simulink model "Demo_veDYNA_cs"  (Simulink 7.6)
settings: Solver=ode1  StartTime=0  StopTime=15  FixedStep=1/500  RelTol=1e-3
model workspace (MAT data in the model file):
  mbox_table : struct (value not decoded)
  model_closed = 0
  sim_status = 0
PreLoadFcn:
  | PreScanveDYNAPreLoadFcn(bdroot);
  | check_NUTS_defined;
  | 
  | assignin('base',['model_closed_' bdroot],false);
PostLoadFcn:
  | PreScanveDYNAPostLoadFcn(bdroot);
  | 
InitFcn:
  | vdy_SetExternalInputSource('ManLongCtrl',1,'Brake','other');
  | vdy_SetExternalInputSource('ManLongCtrl',1,'EngineTorque','other');
  | vdy_SetExternalInputSource('ManLatCtrl',1,'Steering','other');
  | 
  | PreScanveDYNAInitFcn(bdroot);
  | PreScanExperimentInitFcn(bdroot)
StopFcn:
  | PreScanExperimentStopFcn(bdroot)
undefined symbols (not defined in the file): at_period, CPT, vm_at_pulsewidth, vm_driver_dflt_gain, x_ini_VRML, y_ini_VRML, z_ini_VRML
libraries: dyna_cpt_lib x93, simulink x16, simulink_extras x14, PreScanSimulinkLibrary x6, anilib x3, dyna_lib x3, dyna_manctrl_lib x2, dyna_road_lib x2, PreScanUsefulBlocks x1, dyna_io_lib x1, dyna_demo_lib x1, dyna_usr_maneuver_states_lib x1
(part 1 of 8)
CloseFcn:
  | evalin('base',['clear model_closed_' bdroot]);
settings Model: TDMajorMDLVersion=3  TDMinorMDLVersion=3  TDMDLPatchlevel=0  Creator=PRESCAN  LastModifiedBy=cappend  BufferReuse=off
settings OptimizationCC: BlockReduction=off  BooleanDataType=off  ConditionallyExecuteInputs=off  OptimizeBlockIOStorage=off  BufferReuse=off  ExpressionFolding=off  LocalBlockOutputs=off  InitFltsAndDblsToZero=on
settings DebuggingCC: SaveWithParameterizedLinksMsg=none  SignalResolutionControl=TryResolveAllWithWarning  MultiTaskDSMMsg=warning  MultiTaskCondExecSysMsg=none  StrictBusMsg=Warning
settings RTWCC: IncludeERTFirstTime=on
settings GRTTargetCC: TargetFcnLib=ansi_tfl_tmw.mat

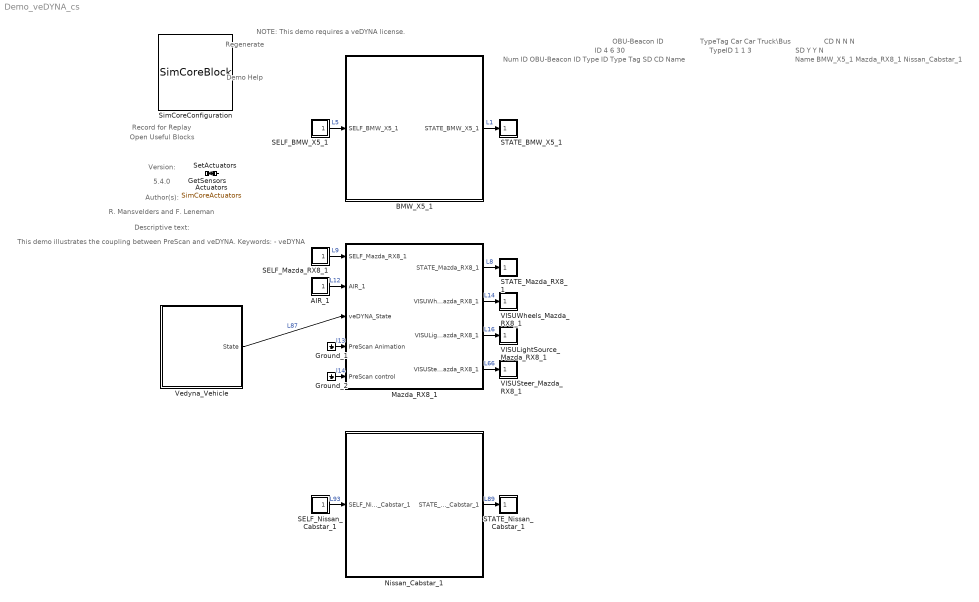
== system Demo_veDYNA_cs ==
  note: Demo Help
  note: NOTE: This demo requires a veDYNA license.
  note: Regenerate
  note: Record for Replay
  note: Open Useful Blocks
  note: Version:
  note: 5.4.0
  note: Author(s):
  note: R. Mansvelders and F. Leneman
  note: Descriptive text:
  note: This demo illustrates the
      | coupling between PreScan and
      | veDYNA.
      |
      | Keywords:
      | - veDYNA
  note: ID
      |
      | 4
      | 6
      | 30
  note: OBU-Beacon ID
  note: TypeID
      |
      | 1
      | 1
      | 3
  note: TypeTag
      |
      | Car
      | Car
      | Truck\Bus
  note: SD
      |
      | Y
      | Y
      | N
  note: CD
      |
      | N
      | N
      | N
  note: Name
      |
      | BMW_X5_1
      | Mazda_RX8_1
      | Nissan_Cabstar_1
  note: Num ID OBU-Beacon ID Type ID Type Tag SD CD Name
  AIR_1 : Subsystem  Tag=AIR  mask(PreScan Source Block: Actor Independent Receiver (AIR)){Angle=60, Range=75, NrEntitiesOut=1, PortName=AIR_1, PortIndex=16, PortWidth=6, TimeStep=1/500}
      mask prompts: Angle "User Specified: Angle [deg]"; Range "User Specified: Range [m]"; NrEntitiesOut "Auto-Assigned: # of Visible Actors in Experiment [-]"; PortName "Auto-Assigned: Port Name [-]"; PortIndex "Auto-Assigned: Port Index [-]"; PortWidth "Auto-Assigned: Port Dimensions [-]"; TimeStep "Auto-Assigned: Upload Period [s]"
      mask help:
      | The Actor Information Receiver sensor provides a fast, simple and generic detection solution which is not tied up to a specific technology. The AIR detects the intersection point of the bounding box with the straight line from the sensor axis system to the middle of the bounding box.
      |
      | For more information, please click Help.
      settings: DeleteFcn=PreScanBlockDeleteFcn;
      mask Help: eval('openHelp(413)')
      mask Display: image(imread('AIR.png'))
  Actuators : DataStoreMemory  Tag=Actuators  DataStoreName=SimCoreActuators  InitialValue=zeros(289,1)
      settings: DeleteFcn=PreScanBlockDeleteFcn;
  BMW_X5_1 : Subsystem  Tag=WorldObjectSubSystem  InitFcn=UniqueId = '15';
      mask Display: image(imread('BMW_X5.jpg'));color('white');text(0,0,' ID=4\n')
  GetSensors : Subsystem  Tag=GetSensors  mask(PreScan Simulation Core Block){NrOfSensors=30, TimeStep=1/500}
      mask prompts: NrOfSensors "Number of sensor values"; TimeStep "Timestep [s]"
      mask help:
      | Please do not remove this block from the PreScan compilation sheet,
      | as it contains essential configuration parameters for a PreScan simulation.
      settings: DeleteFcn=PreScanBlockDeleteFcn;
  Ground_1 : Ground
  Ground_2 : Ground
  Mazda_RX8_1 : Subsystem  Tag=WorldObjectSubSystem  InitFcn=UniqueId = '17';
      mask Display: image(imread('Mazda_RX8.jpg'));color('white');text(0,0,' ID=6\n')
  Nissan_Cabstar_1 : Subsystem  Tag=WorldObjectSubSystem  InitFcn=UniqueId = '45';
      mask Display: image(imread('Nissan_Cabstar.jpg'));color('white');text(0,0,' ID=30\n')
  SELF_BMW_X5_1 : Subsystem  Tag=SELF  mask(PreScan Source Block: SELF){PortName=SELF_BMW_X5_1, PortIndex=0, PortWidth=8, TimeStep=1/500}
      mask prompts: PortName "Auto-Assigned: Port Name [-]"; PortIndex "Auto-Assigned: Port Index [-]"; PortWidth "Auto-Assigned: Port Dimensions"; TimeStep "Auto-Assigned: Upload Period [s]"
      mask help:
      | The SELF port shows (state) information of the actor itself. The outputs are position in the experiment's axis system and the GPS coordinates, and the object's absolute velocity and compass heading.
      |
      | For more information, please click Help.
      settings: DeleteFcn=PreScanBlockDeleteFcn;
      mask Help: eval('openHelp(462)')
      mask Display: image(imread('GPS.png'))
  SELF_Mazda_RX8_1 : Subsystem  Tag=SELF  mask(PreScan Source Block: SELF){PortName=SELF_Mazda_RX8_1, PortIndex=8, PortWidth=8, TimeStep=1/500}
      mask prompts: PortName "Auto-Assigned: Port Name [-]"; PortIndex "Auto-Assigned: Port Index [-]"; PortWidth "Auto-Assigned: Port Dimensions"; TimeStep "Auto-Assigned: Upload Period [s]"
      mask help:
      | The SELF port shows (state) information of the actor itself. The outputs are position in the experiment's axis system and the GPS coordinates, and the object's absolute velocity and compass heading.
      |
      | For more information, please click Help.
      settings: DeleteFcn=PreScanBlockDeleteFcn;
      mask Help: eval('openHelp(462)')
      mask Display: image(imread('GPS.png'))
  SELF_Nissan_Cabstar_1 : Subsystem  Tag=SELF  mask(PreScan Source Block: SELF){PortName=SELF_Nissan_Cabstar_1, PortIndex=22, PortWidth=8, TimeStep=1/500}
      mask prompts: PortName "Auto-Assigned: Port Name [-]"; PortIndex "Auto-Assigned: Port Index [-]"; PortWidth "Auto-Assigned: Port Dimensions"; TimeStep "Auto-Assigned: Upload Period [s]"
      mask help:
      | The SELF port shows (state) information of the actor itself. The outputs are position in the experiment's axis system and the GPS coordinates, and the object's absolute velocity and compass heading.
      |
      | For more information, please click Help.
      settings: DeleteFcn=PreScanBlockDeleteFcn;
      mask Help: eval('openHelp(462)')
      mask Display: image(imread('GPS.png'))
  STATE_BMW_X5_1 : Subsystem  Tag=State  mask(PreScan Sink Block: State){x0=10.1045246, y0=47.3258, z0=0.69, Roll0=0, Pitch0=0, Yaw0=0, override=off, Mode=Positioning}
      mask prompts: x0 "Ini x-position VEHICLE wrt GLOBAL axis system [m]"; y0 "Ini y-position VEHICLE wrt GLOBAL axis system [m]"; z0 "Ini z-position VEHICLE wrt GLOBAL axis system [m]"; Roll0 "Ini roll-angle BODY wrt VEHICLE axis system [rad]"; Pitch0 "Ini pitch-angle BODY wrt VEHICLE axis system [rad]"; Yaw0 "Ini yaw-angle VEHICLE wrt GLOBAL axis system [rad]"; override "Override Mode"
      mask help:
      | The Actor State contains a vector signal of size (9x1), containing the following signals:
      |
      | -  Position                  (x,y,z)                                     [m]
      | -  Velocity                  (vx,vy,vz)                               [m/s]
      | -  Angles                    (Roll, Pitch, Yaw)                   [rad]
      |
      | The Actor state is defined in the global axis system.
      | The state is superponed on the Initial position defined in the GUI.
      |
      | For more information, please click Help.
      settings: DeleteFcn=PreScanBlockDeleteFcn;
      mask Help: eval('openHelp(222)')
      mask StyleString: edit,edit,edit,edit,edit,edit,checkbox,popup(Positioning|Dynamics)
      mask CallbackString: ||||||StateOverrideFcn('General')|
      mask Display: image(imread('State.png'))
  STATE_Mazda_RX8_1 : Subsystem  Tag=State  mask(PreScan Sink Block: State){x0=-9.892563, y0=51.9277153, z0=0.51, Roll0=0, Pitch0=0, Yaw0=0, override=on, Mode=Positioning}
      mask prompts: x0 "Ini x-position VEHICLE wrt GLOBAL axis system [m]"; y0 "Ini y-position VEHICLE wrt GLOBAL axis system [m]"; z0 "Ini z-position VEHICLE wrt GLOBAL axis system [m]"; Roll0 "Ini roll-angle BODY wrt VEHICLE axis system [rad]"; Pitch0 "Ini pitch-angle BODY wrt VEHICLE axis system [rad]"; Yaw0 "Ini yaw-angle VEHICLE wrt GLOBAL axis system [rad]"; override "Override Mode"
      mask help:
      | The Actor State contains a vector signal of size (9x1), containing the following signals:
      |
      | -  Position                  (x,y,z)                                     [m]
      | -  Velocity                  (vx,vy,vz)                               [m/s]
      | -  Angles                    (Roll, Pitch, Yaw)                   [rad]
      |
      | The Actor state is defined in the global axis system.
      | The state is superponed on the Initial position defined in the GUI.
      |
      | For more information, please click Help.
      settings: DeleteFcn=PreScanBlockDeleteFcn;
      mask Help: eval('openHelp(222)')
      mask StyleString: edit,edit,edit,edit,edit,edit,checkbox,popup(Positioning|Dynamics)
      mask CallbackString: ||||||StateOverrideFcn('General')|
      mask Display: image(imread('State.png'))
  STATE_Nissan_Cabstar_1 : Subsystem  Tag=State  mask(PreScan Sink Block: State){x0=-14, y0=47.3258, z0=0.88, Roll0=0, Pitch0=0, Yaw0=0, override=off, Mode=Positioning}
      mask prompts: x0 "Ini x-position VEHICLE wrt GLOBAL axis system [m]"; y0 "Ini y-position VEHICLE wrt GLOBAL axis system [m]"; z0 "Ini z-position VEHICLE wrt GLOBAL axis system [m]"; Roll0 "Ini roll-angle BODY wrt VEHICLE axis system [rad]"; Pitch0 "Ini pitch-angle BODY wrt VEHICLE axis system [rad]"; Yaw0 "Ini yaw-angle VEHICLE wrt GLOBAL axis system [rad]"; override "Override Mode"
      mask help:
      | The Actor State contains a vector signal of size (9x1), containing the following signals:
      |
      | -  Position                  (x,y,z)                                     [m]
      | -  Velocity                  (vx,vy,vz)                               [m/s]
      | -  Angles                    (Roll, Pitch, Yaw)                   [rad]
      |
      | The Actor state is defined in the global axis system.
      | The state is superponed on the Initial position defined in the GUI.
      |
      | For more information, please click Help.
      settings: DeleteFcn=PreScanBlockDeleteFcn;
      mask Help: eval('openHelp(222)')
      mask StyleString: edit,edit,edit,edit,edit,edit,checkbox,popup(Positioning|Dynamics)
      mask CallbackString: ||||||StateOverrideFcn('General')|
      mask Display: image(imread('State.png'))
  SetActuators : Subsystem  Tag=SetActuators  mask(PreScan Simulation Core Block){TimeStep=1/500, NrOfActuators=289}
      mask prompts: TimeStep "Timestep [s]"; NrOfActuators "Number of actuator values"
      mask help:
      | Please do not remove this block from the PreScan compilation sheet,
      | as it contains essential configuration parameters for a PreScan simulation.
      settings: DeleteFcn=PreScanBlockDeleteFcn;
  SimCoreConfiguration : M-S-Function  Tag=SimCoreConfiguration  Description=A17A9ED9750FB4A86C3BBE414AD268275C76F333D22CB9730EAC2D9853BCC9CB  FunctionName=SimCoreBlock  Parameters=ExperimentXML PortsXML SimulationCore HostName CheckStart EnableLog RfR  mask(PreScan Simulation Core Configurator){SimulationCore=NUTS, HostName=0, CheckStart=0, prescanversion='5.4.0', EnableLog=off, RfR=0}
      mask prompts: SimulationCore "Simulation Core"; HostName "Simulation Host"; CheckStart "Show START Dialog"; prescanversion "PreScan Version"; EnableLog "Create TA Log"; RfR "Record for Replay"
      mask help:
      | Please do not remove this block from the PreScan compilation sheet,
      | as it contains essential configuration parameter for a PreScan simulation.
      mask init:
      | model = bdroot;
      | ExperimentXML = [model(1:end-3) '.pex'];
      | PortsXML = [model '_ports.pcd'];
      settings: DeleteFcn=PreScanBlockDeleteFcn;  ModelCloseFcn=assignin('base',['model_closed_' bdroot],true);
      mask Display: image(imread('prescanlogo.ico'))
  VISULightSource_Mazda_RX8_1 : Subsystem  Tag=VisuLightSource
      settings: DeleteFcn=PreScanBlockDeleteFcn;
      mask Type: PreScan Sink Block: VisuLightSource
      mask Description:
      | The VisuLightSource block provides a way to animate Light Sources of the indicator, braking, fog and main lights of a vehicle.
      | 
      | For more information, please click Help.
      mask Help: eval('openHelp(223)')
      mask Display: image(imread('RearLight.png'))
  VISUSteer_Mazda_RX8_1 : Subsystem  Tag=VisuSteer
      settings: DeleteFcn=PreScanBlockDeleteFcn;
      mask Type: PreScan Sink Block: VisuSteer
      mask Description:
      | The VisuSteer block provides a way to adapt the orientation of the steering column and steering wheel of a vehicle.
      | 
      | For more information, please click Help.
      mask Help: eval('openHelp(223)')
      mask Display: image(imread('steeringwheel.png'))
  VISUWheels_Mazda_RX8_1 : Subsystem  Tag=VisuWheels
      settings: DeleteFcn=PreScanBlockDeleteFcn;
      mask Type: PreScan Sink Block: VisuWheels
      mask Description:
      | The VisuWheels block provides a way to animate the wheels of a vehicle, with steering, rotation (because of velocity) and z-displacement.
      | 
      | For more information, please click Help.
      mask Help: eval('openHelp(223)')
      mask Display: image(imread('wheel.png'))
  Vedyna_Vehicle : Subsystem  Tag=UserSpecified_Subsys  Description=C:\Program Files\DYNAwareR3.3\work.current\models\vedyna_vehicle.mdl  mask(User specified subsystem){update=off, sourcefilename=C:\\Program Files\\DYNAwareR3.3\\work.current\\models\\vedyna_vehicle.mdl}
      mask prompts: update "Update (default: not checked)"; sourcefilename "Source file name"
      mask help:
      | A User-specified model may be selected as Controller or Dynamics of the vehicle. PreScan will copy the contents of the User-specified model into the user-specified model block.
      |
      | If update checkbox is checked the current user-specified model block will be deleted and will be REPLACED by (new) user specified model blocks. So, the current user specified model elements will be lost.
      |
      | Warning: If a new user-specified model is selected in the GUI, the user-specified model will be replaced.
      settings: DeleteFcn=PreScanBlockDeleteFcn;
      mask Help: eval('openHelp(227)')
      mask Display:
      | image(imread('UserSpecDyn.png'))
      | port_label('output', 1, 'State'); text(0,0,' veDYNA Vehicle\n')
  wires:
  SetActuators/1(dummy) -> GetSensors/1(dummy)
  BMW_X5_1/1(STATE_BMW_X5_1) -> STATE_BMW_X5_1/1(State)  "L1"
  SELF_BMW_X5_1/1(U) -> BMW_X5_1/1(SELF_BMW_X5_1)  "L5"
  Mazda_RX8_1/1(STATE_Mazda_RX8_1) -> STATE_Mazda_RX8_1/1(State)  "L8"
  SELF_Mazda_RX8_1/1(U) -> Mazda_RX8_1/1(SELF_Mazda_RX8_1)  "L9"
  AIR_1/1(U) -> Mazda_RX8_1/2(AIR_1)  "L12"
  Mazda_RX8_1/2(VISUWheels_Mazda_RX8_1) -> VISUWheels_Mazda_RX8_1/1(Wheels)  "L14"
  Mazda_RX8_1/3(VISULightSource_Mazda_RX8_1) -> VISULightSource_Mazda_RX8_1/1(Lights)  "L16"
  Mazda_RX8_1/4(VISUSteer_Mazda_RX8_1) -> VISUSteer_Mazda_RX8_1/1(Steer)  "L66"
  Vedyna_Vehicle/1(State) -> Mazda_RX8_1/3(veDYNA_State)  "L87"
  Nissan_Cabstar_1/1(STATE_Nissan_Cabstar_1) -> STATE_Nissan_Cabstar_1/1(State)  "L89"
  SELF_Nissan_Cabstar_1/1(U) -> Nissan_Cabstar_1/1(SELF_Nissan_Cabstar_1)  "L93"
  Ground_1/1 -> Mazda_RX8_1/4(PreScan Animation)  "l13"
  Ground_2/1 -> Mazda_RX8_1/5(PreScan control)  "l14"

== system Demo_veDYNA_cs/AIR_1 ==
  Selector : Selector  IndexMode=Zero-based  IndexOptions=Starting index (dialog)  Indices=PortIndex  OutputSizes=PortWidth(1)
  U : Outport
  wires:
  Selector/1 -> U/1
  [SimCoreSensors] -> Selector/1

== system Demo_veDYNA_cs/BMW_X5_1 ==
  SELF_BMW_X5_1 : Inport  Tag=SELFInport
  SELF_Demux : Subsystem  Tag=DemuxSELF
      settings: DeleteFcn=PreScanBlockDeleteFcn;
      mask Type: PreScan Demux Block:
      mask Display:
      | port_label('output',1,'x [m]')
      | port_label('output',2,'y [m]')
      | port_label('output',3,'z [m]','texmode','on')
      | port_label('output',4,'Rotx [deg]','texmode','on')
      | port_label('output',5,'Roty [deg]','texmode','on')
      | port_label('output',6,'Rotz [deg]','texmode','on')
      | port_label('output',7,'GPS lat [deg]','texmode','on')
      | port_label('output',8,'GPS long [deg]','texmode','on')
      | port_label('output',9,'GPS alt [m]','texmode','on')
      | port_label('output',10,'Velocity [m/s]')
      | port_label('output',11,'Heading [deg]')
      | port_label('output',12,'Yaw rate [deg/s]')
  Terminator_{1..12} (12 alike) : Terminator
  Trajectories : Subsystem  Tag=Trajectories
      settings: DeleteFcn=PreScanBlockDeleteFcn;
      mask Display: image(imread('Trajectory.png'));
  STATE_BMW_X5_1 : Outport  Tag=StateOutport
  wires:
  SELF_BMW_X5_1/1 -> SELF_Demux/1(SELF)  "L6"
  Trajectories/1(State) -> STATE_BMW_X5_1/1  "L7"
  SELF_Demux/1(x [m]) -> Terminator_1/1  "l1"
  SELF_Demux/2(y [m]) -> Terminator_2/1  "l2"
  SELF_Demux/3(z [m]) -> Terminator_3/1  "l3"
  SELF_Demux/4(rotx [deg]) -> Terminator_4/1  "l4"
  SELF_Demux/5(roty [deg]) -> Terminator_5/1  "l5"
  SELF_Demux/6(rotz [deg]) -> Terminator_6/1  "l6"
  SELF_Demux/7(GPS lat [deg]) -> Terminator_7/1  "l7"
  SELF_Demux/8(GPS long [deg]) -> Terminator_8/1  "l8"
  SELF_Demux/9(GPS alt [m]) -> Terminator_9/1  "l9"
  SELF_Demux/10(velocity [m/s]) -> Terminator_10/1  "l10"
  SELF_Demux/11(heading [deg]) -> Terminator_11/1  "l11"
  SELF_Demux/12(yaw rate [deg/s]) -> Terminator_12/1  "l12"

== system Demo_veDYNA_cs/GetSensors ==
  dummy : Inport
  GetSensors : M-S-Function  FunctionName=GetSensorsBlock  Parameters=TimeStep, NrOfSensors
      mask Type: PreScan GetSensors block
      mask Description: Reads new sensor values from the simulation core
  tag scope: SimCoreSensors=global
  wires:
  GetSensors/1 -> [SimCoreSensors]
  dummy/1 -> GetSensors/1

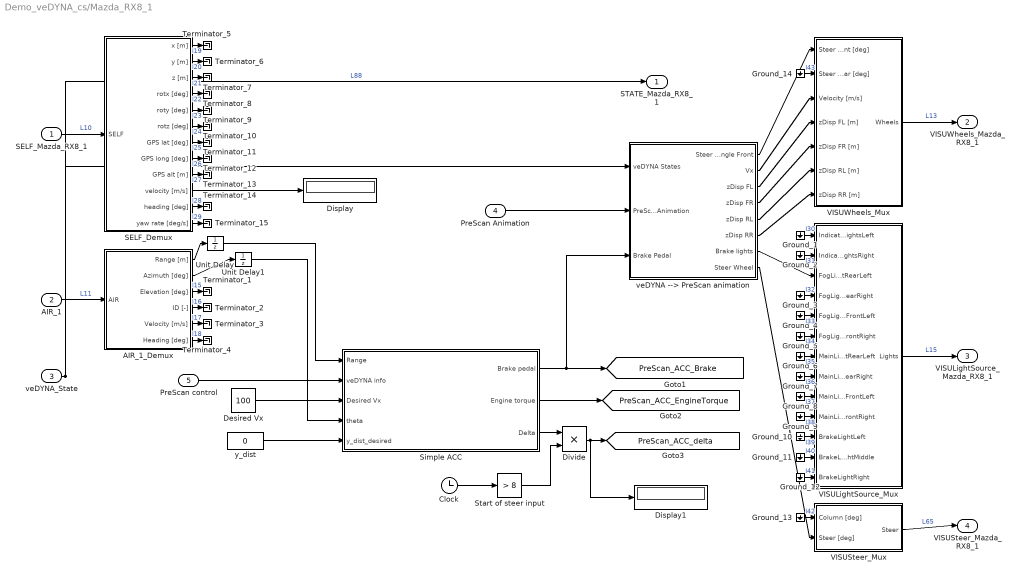
== system Demo_veDYNA_cs/Mazda_RX8_1 ==
  SELF_Mazda_RX8_1 : Inport  Tag=SELFInport
  AIR_1 : Inport  Tag=AIRInport  Port=2
  veDYNA_State : Inport  Tag=veDYNA_StateInport  Port=3
  PreScan Animation : Inport  Tag=AIRInport  Port=4
  PreScan control : Inport  Tag=AIRInport  Port=5
  AIR_1_Demux : Subsystem  Tag=DemuxAIR  mask(PreScan Demux Block:){DetectionType=BBox}
      mask prompts: DetectionType "Detection Type"
      mask init:
      | switch DetectionType
      |     case 1
      |         DetectionTypeStr = 'Shortest';
      |     case 2
      |         DetectionTypeStr = 'BBox';
      |     case 3
      |         DetectionTypeStr = 'CoG';
      |     otherwise
      |         DetectionTypeStr = 'Unknown';
      | end
      settings: DeleteFcn=PreScanBlockDeleteFcn;
      mask StyleString: popup(Shortest|BBox|CoG)
      mask Display:
      | disp(char('Det. type:         ',['{\it',DetectionTypeStr,'}']),'texmode','on')
      | port_label('output',1,'Range [m]')
      | port_label('output',2,'{\theta} [deg]','texmode','on')
      | port_label('output',3,'{\phi} [deg]','texmode','on')
      | port_label('output',4,'ID [-]','texmode','on')
      | port_label('output',5,'Velocity [m/s]','texmode','on')
      | port_label('output',6,'Heading [deg]','texmode','on')
  Clock : Clock
      settings: Decimation=10
  Desired Vx : Constant  Value=100
  Display : Display
  Display1 : Display
  Divide : Product  Inputs=**
  Ground_{1..14} (14 alike) : Ground
  SELF_Demux : Subsystem  Tag=DemuxSELF
      settings: DeleteFcn=PreScanBlockDeleteFcn;
      mask Type: PreScan Demux Block:
      mask Display:
      | port_label('output',1,'x [m]')
      | port_label('output',2,'y [m]')
      | port_label('output',3,'z [m]','texmode','on')
      | port_label('output',4,'Rotx [deg]','texmode','on')
      | port_label('output',5,'Roty [deg]','texmode','on')
      | port_label('output',6,'Rotz [deg]','texmode','on')
      | port_label('output',7,'GPS lat [deg]','texmode','on')
      | port_label('output',8,'GPS long [deg]','texmode','on')
      | port_label('output',9,'GPS alt [m]','texmode','on')
      | port_label('output',10,'Velocity [m/s]')
      | port_label('output',11,'Heading [deg]')
      | port_label('output',12,'Yaw rate [deg/s]')
  Simple ACC : Subsystem
  Start of steer input : simulink/Logic and Bit Operations/Compare To Constant  SystemSampleTime=-1  relop=>  const=8  LogicOutDataTypeMode=uint8  ZeroCross=off
  Terminator_{1..15} (15 alike) : Terminator
  Unit Delay : UnitDelay  SampleTime=-1
  Unit Delay1 : UnitDelay  SampleTime=-1
  VISULightSource_Mux : Subsystem  Tag=MuxLightSource
      settings: DeleteFcn=PreScanBlockDeleteFcn;
      mask Type: PreScan Mux Block:
  VISUSteer_Mux : Subsystem  Tag=MuxSteer
      settings: DeleteFcn=PreScanBlockDeleteFcn;
      mask Type: PreScan Mux Block:
  VISUWheels_Mux : Subsystem  Tag=MuxWheels
      settings: DeleteFcn=PreScanBlockDeleteFcn;
      mask Type: PreScan Mux Block:
  veDYNA --> PreScan animation : Subsystem
  y_dist : Constant  Value=0
  STATE_Mazda_RX8_1 : Outport  Tag=StateOutport
  VISUWheels_Mazda_RX8_1 : Outport  Tag=VisuWheelsOutport  Port=2
  VISULightSource_Mazda_RX8_1 : Outport  Tag=VisuLightsOutport  Port=3
  VISUSteer_Mazda_RX8_1 : Outport  Tag=VisuSteerOutport  Port=4
  tag scope: PreScan_ACC_Brake=global, PreScan_ACC_EngineTorque=global, PreScan_ACC_delta=global
  wires:
  Desired Vx/1 -> Simple ACC/3(Desired Vx)
  y_dist/1 -> Simple ACC/5(y_dist_desired)
  Simple ACC/3(Delta) -> Divide/1
  Simple ACC/1(Brake pedal) -> [PreScan_ACC_Brake], veDYNA --> PreScan animation/3(Brake Pedal)
  Simple ACC/2(Engine torque) -> [PreScan_ACC_EngineTorque]
  Unit Delay/1 -> Simple ACC/1(Range)
  Unit Delay1/1 -> Simple ACC/4(theta)
  Divide/1 -> [PreScan_ACC_delta], Display1/1
  Clock/1 -> Start of steer input/1
  Start of steer input/1 -> Divide/2
  veDYNA_State/1 -> veDYNA --> PreScan animation/1(veDYNA States), STATE_Mazda_RX8_1/1  "L88"
  veDYNA --> PreScan animation/8(Steer Wheel) -> VISUSteer_Mux/2(Steer [deg])
  AIR_1_Demux/1(Range [m]) -> Unit Delay/1
  AIR_1_Demux/2(Azimuth [deg]) -> Unit Delay1/1
  PreScan control/1 -> Simple ACC/2(veDYNA info)
  SELF_Demux/10(velocity [m/s]) -> Display/1
  PreScan Animation/1 -> veDYNA --> PreScan animation/2(PreScan Animation)
  veDYNA --> PreScan animation/1(Steer Angle Front) -> VISUWheels_Mux/1(Steer Angle Front [deg])
  veDYNA --> PreScan animation/2(Vx) -> VISUWheels_Mux/3(Velocity [m/s])
  veDYNA --> PreScan animation/3(zDisp FL) -> VISUWheels_Mux/4(zDisp FL [m])
  veDYNA --> PreScan animation/4(zDisp FR) -> VISUWheels_Mux/5(zDisp FR [m])
  veDYNA --> PreScan animation/5(zDisp RL) -> VISUWheels_Mux/6(zDisp RL [m])
  veDYNA --> PreScan animation/6(zDisp RR) -> VISUWheels_Mux/7(zDisp RR [m])
  veDYNA --> PreScan animation/7(Brake lights) -> VISULightSource_Mux/3(FogLightRearLeft)
  SELF_Mazda_RX8_1/1 -> SELF_Demux/1(SELF)  "L10"
  AIR_1/1 -> AIR_1_Demux/1(AIR)  "L11"
  VISUWheels_Mux/1(Wheels) -> VISUWheels_Mazda_RX8_1/1  "L13"
  VISULightSource_Mux/1(Lights) -> VISULightSource_Mazda_RX8_1/1  "L15"
  VISUSteer_Mux/1(Steer) -> VISUSteer_Mazda_RX8_1/1  "L65"
  AIR_1_Demux/3(Elevation [deg]) -> Terminator_1/1  "l15"
  AIR_1_Demux/4(ID [-]) -> Terminator_2/1  "l16"
  AIR_1_Demux/5(Velocity [m/s]) -> Terminator_3/1  "l17"
  AIR_1_Demux/6(Heading [deg]) -> Terminator_4/1  "l18"
  SELF_Demux/1(x [m]) -> Terminator_5/1  "l19"
  SELF_Demux/2(y [m]) -> Terminator_6/1  "l20"
  SELF_Demux/3(z [m]) -> Terminator_7/1  "l21"
  SELF_Demux/4(rotx [deg]) -> Terminator_8/1  "l22"
  SELF_Demux/5(roty [deg]) -> Terminator_9/1  "l23"
  SELF_Demux/6(rotz [deg]) -> Terminator_10/1  "l24"
  SELF_Demux/7(GPS lat [deg]) -> Terminator_11/1  "l25"
  SELF_Demux/8(GPS long [deg]) -> Terminator_12/1  "l26"
  SELF_Demux/9(GPS alt [m]) -> Terminator_13/1  "l27"
  SELF_Demux/11(heading [deg]) -> Terminator_14/1  "l28"
  SELF_Demux/12(yaw rate [deg/s]) -> Terminator_15/1  "l29"
  Ground_1/1 -> VISULightSource_Mux/1(IndicatorLightsLeft)  "l30"
  Ground_2/1 -> VISULightSource_Mux/2(IndicatorLightsRight)  "l31"
  Ground_3/1 -> VISULightSource_Mux/4(FogLightRearRight)  "l32"
  Ground_4/1 -> VISULightSource_Mux/5(FogLightFrontLeft)  "l33"
  Ground_5/1 -> VISULightSource_Mux/6(FogLightFrontRight)  "l34"
  Ground_6/1 -> VISULightSource_Mux/7(MainLightRearLeft)  "l35"
  Ground_7/1 -> VISULightSource_Mux/8(MainLightRearRight)  "l36"
  Ground_8/1 -> VISULightSource_Mux/9(MainLightFrontLeft)  "l37"
  Ground_9/1 -> VISULightSource_Mux/10(MainLightFrontRight)  "l38"
  Ground_10/1 -> VISULightSource_Mux/11(BrakeLightLeft)  "l39"
  Ground_11/1 -> VISULightSource_Mux/12(BrakeLightMiddle)  "l40"
  Ground_12/1 -> VISULightSource_Mux/13(BrakeLightRight)  "l41"
  Ground_13/1 -> VISUSteer_Mux/1(Column [deg])  "l42"
  Ground_14/1 -> VISUWheels_Mux/2(Steer Angle Rear [deg])  "l43"

== system Demo_veDYNA_cs/Nissan_Cabstar_1 ==
  SELF_Nissan_Cabstar_1 : Inport  Tag=SELFInport
  SELF_Demux : Subsystem  Tag=DemuxSELF
      settings: DeleteFcn=PreScanBlockDeleteFcn;
      mask Type: PreScan Demux Block:
      mask Display:
      | port_label('output',1,'x [m]')
      | port_label('output',2,'y [m]')
      | port_label('output',3,'z [m]','texmode','on')
      | port_label('output',4,'Rotx [deg]','texmode','on')
      | port_label('output',5,'Roty [deg]','texmode','on')
      | port_label('output',6,'Rotz [deg]','texmode','on')
      | port_label('output',7,'GPS lat [deg]','texmode','on')
      | port_label('output',8,'GPS long [deg]','texmode','on')
      | port_label('output',9,'GPS alt [m]','texmode','on')
      | port_label('output',10,'Velocity [m/s]')
      | port_label('output',11,'Heading [deg]')
      | port_label('output',12,'Yaw rate [deg/s]')
  Terminator_{1..12} (12 alike) : Terminator
  Trajectories : Subsystem  Tag=Trajectories
      settings: DeleteFcn=PreScanBlockDeleteFcn;
      mask Display: image(imread('Trajectory.png'));
  STATE_Nissan_Cabstar_1 : Outport  Tag=StateOutport
  wires:
  SELF_Nissan_Cabstar_1/1 -> SELF_Demux/1(SELF)  "L94"
  Trajectories/1(State) -> STATE_Nissan_Cabstar_1/1  "L95"
  SELF_Demux/1(x [m]) -> Terminator_1/1  "l44"
  SELF_Demux/2(y [m]) -> Terminator_2/1  "l45"
  SELF_Demux/3(z [m]) -> Terminator_3/1  "l46"
  SELF_Demux/4(rotx [deg]) -> Terminator_4/1  "l47"
  SELF_Demux/5(roty [deg]) -> Terminator_5/1  "l48"
  SELF_Demux/6(rotz [deg]) -> Terminator_6/1  "l49"
  SELF_Demux/7(GPS lat [deg]) -> Terminator_7/1  "l50"
  SELF_Demux/8(GPS long [deg]) -> Terminator_8/1  "l51"
  SELF_Demux/9(GPS alt [m]) -> Terminator_9/1  "l52"
  SELF_Demux/10(velocity [m/s]) -> Terminator_10/1  "l53"
  SELF_Demux/11(heading [deg]) -> Terminator_11/1  "l54"
  SELF_Demux/12(yaw rate [deg/s]) -> Terminator_12/1  "l55"

== system Demo_veDYNA_cs/SELF_BMW_X5_1 ==
  Selector : Selector  IndexMode=Zero-based  IndexOptions=Starting index (dialog)  Indices=PortIndex  OutputSizes=PortWidth(1)
  U : Outport
  wires:
  Selector/1 -> U/1
  [SimCoreSensors] -> Selector/1

== system Demo_veDYNA_cs/SELF_Mazda_RX8_1 ==
  Selector : Selector  IndexMode=Zero-based  IndexOptions=Starting index (dialog)  Indices=PortIndex  OutputSizes=PortWidth(1)
  U : Outport
  wires:
  Selector/1 -> U/1
  [SimCoreSensors] -> Selector/1

== system Demo_veDYNA_cs/SELF_Nissan_Cabstar_1 ==
  Selector : Selector  IndexMode=Zero-based  IndexOptions=Starting index (dialog)  Indices=PortIndex  OutputSizes=PortWidth(1)
  U : Outport
  wires:
  Selector/1 -> U/1
  [SimCoreSensors] -> Selector/1

== system Demo_veDYNA_cs/STATE_BMW_X5_1 ==
  State : Inport
  Acceleration : Subsystem  mask(ToSensorWorld){PortName=Acceleration_BMW_X5_1, PortIndex=6, PortWidth=3, TimeStep=1/500}
      mask prompts: PortName "Port Name [-]"; PortIndex "Index [-]"; PortWidth "Port Dimensions [-]"; TimeStep "Upload Period [s]"
      mask help: Sends signal(s) from Simulink to the Sensor World
      mask Help:
      | Sends signal(s) from Simulink to the Sensor World.
      | 
      | - Port Name [-]: specifies the name of the output terminal of the Simulink block.
      | - Index [-]: specifies the start position in the output vector sent to the Sensor World
      | - Port dimensions [-]: specifies the width (number of scalars) of the output port
      | - Upload period [s]: specifies the upload period (in seconds) of the port.
      mask Display: port_label('input', 1, PortName)
  Demux : Demux  Outputs=5
  Position : Subsystem  mask(ToSensorWorld){PortName=Position_BMW_X5_1, PortIndex=0, PortWidth=3, TimeStep=1/500}
      mask prompts: PortName "Port Name [-]"; PortIndex "Index [-]"; PortWidth "Port Dimensions [-]"; TimeStep "Upload Period [s]"
      mask help: Sends signal(s) from Simulink to the Sensor World
      mask Help:
      | Sends signal(s) from Simulink to the Sensor World.
      | 
      | - Port Name [-]: specifies the name of the output terminal of the Simulink block.
      | - Index [-]: specifies the start position in the output vector sent to the Sensor World
      | - Port dimensions [-]: specifies the width (number of scalars) of the output port
      | - Upload period [s]: specifies the upload period (in seconds) of the port.
      mask Display: port_label('input', 1, PortName)
  RPY : Subsystem  mask(ToSensorWorld){PortName=RPY_BMW_X5_1, PortIndex=9, PortWidth=3, TimeStep=1/500}
      mask prompts: PortName "Port Name [-]"; PortIndex "Index [-]"; PortWidth "Port Dimensions [-]"; TimeStep "Upload Period [s]"
      mask help: Sends signal(s) from Simulink to the Sensor World
      mask Help:
      | Sends signal(s) from Simulink to the Sensor World.
      | 
      | - Port Name [-]: specifies the name of the output terminal of the Simulink block.
      | - Index [-]: specifies the start position in the output vector sent to the Sensor World
      | - Port dimensions [-]: specifies the width (number of scalars) of the output port
      | - Upload period [s]: specifies the upload period (in seconds) of the port.
      mask Display: port_label('input', 1, PortName)
  Velocity : Subsystem  mask(ToSensorWorld){PortName=Velocity_BMW_X5_1, PortIndex=3, PortWidth=3, TimeStep=1/500}
      mask prompts: PortName "Port Name [-]"; PortIndex "Index [-]"; PortWidth "Port Dimensions [-]"; TimeStep "Upload Period [s]"
      mask help: Sends signal(s) from Simulink to the Sensor World
      mask Help:
      | Sends signal(s) from Simulink to the Sensor World.
      | 
      | - Port Name [-]: specifies the name of the output terminal of the Simulink block.
      | - Index [-]: specifies the start position in the output vector sent to the Sensor World
      | - Port dimensions [-]: specifies the width (number of scalars) of the output port
      | - Upload period [s]: specifies the upload period (in seconds) of the port.
      mask Display: port_label('input', 1, PortName)
  iniBODYAngles wrtVEH [rad] : Constant  Value=[Roll0 Pitch0 0]
  iniVEHAngles wrtGLOB [rad] : Constant  Value=[0 0 Yaw0]
  iniVEHposition wrtGLOB [m] : Constant  Value=[x0 y0 z0]
  state2FullState : Subsystem  mask(PreScan Demux Block:){Mode=Mode}
      mask prompts: Mode "Mask Parameter 1:"
      mask init:
      | if strcmp(Mode,'Positioning')
      |     SwitchMode=1;
      | else
      |     SwitchMode=0;
      | end
      | 
      | set_param([gcb,'/SwitchMode'],'sw',num2str(SwitchMode));
      | set_param([gcb,'/SwitchMode1'],'sw',num2str(SwitchMode));
      mask Display: disp(Mode)
  velRPY : Subsystem  mask(ToSensorWorld){PortName=velRPY_BMW_X5_1, PortIndex=12, PortWidth=3, TimeStep=1/500}
      mask prompts: PortName "Port Name [-]"; PortIndex "Index [-]"; PortWidth "Port Dimensions [-]"; TimeStep "Upload Period [s]"
      mask help: Sends signal(s) from Simulink to the Sensor World
      mask Help:
      | Sends signal(s) from Simulink to the Sensor World.
      | 
      | - Port Name [-]: specifies the name of the output terminal of the Simulink block.
      | - Index [-]: specifies the start position in the output vector sent to the Sensor World
      | - Port dimensions [-]: specifies the width (number of scalars) of the output port
      | - Upload period [s]: specifies the upload period (in seconds) of the port.
      mask Display: port_label('input', 1, PortName)
  wires:
  iniVEHAngles wrtGLOB [rad]/1 -> state2FullState/4(iniVEH Angles wrt GLOB axis system [deg])
  iniBODYAngles wrtVEH [rad]/1 -> state2FullState/3(iniBODY Angles wrt VEH axis system [deg])
  iniVEHposition wrtGLOB [m]/1 -> state2FullState/2(ini VEHpos wrt GLOB axis system  [m])
  state2FullState/1(State) -> Demux/1
  State/1 -> state2FullState/1(dx,dy,dz [m/s] R,P,Y  [rad])
  Demux/1 -> Position/1(Y)
  Demux/2 -> Velocity/1(Y)
  Demux/3 -> Acceleration/1(Y)
  Demux/4 -> RPY/1(Y)
  Demux/5 -> velRPY/1(Y)

== system Demo_veDYNA_cs/STATE_Mazda_RX8_1 ==
  State : Inport
  Acceleration : Subsystem  mask(ToSensorWorld){PortName=Acceleration_Mazda_RX8_1, PortIndex=21, PortWidth=3, TimeStep=1/500}
      mask prompts: PortName "Port Name [-]"; PortIndex "Index [-]"; PortWidth "Port Dimensions [-]"; TimeStep "Upload Period [s]"
      mask help: Sends signal(s) from Simulink to the Sensor World
      mask Help:
      | Sends signal(s) from Simulink to the Sensor World.
      | 
      | - Port Name [-]: specifies the name of the output terminal of the Simulink block.
      | - Index [-]: specifies the start position in the output vector sent to the Sensor World
      | - Port dimensions [-]: specifies the width (number of scalars) of the output port
      | - Upload period [s]: specifies the upload period (in seconds) of the port.
      mask Display: port_label('input', 1, PortName)
  Demux : Demux  Outputs=5
  Position : Subsystem  mask(ToSensorWorld){PortName=Position_Mazda_RX8_1, PortIndex=15, PortWidth=3, TimeStep=1/500}
      mask prompts: PortName "Port Name [-]"; PortIndex "Index [-]"; PortWidth "Port Dimensions [-]"; TimeStep "Upload Period [s]"
      mask help: Sends signal(s) from Simulink to the Sensor World
      mask Help:
      | Sends signal(s) from Simulink to the Sensor World.
      | 
      | - Port Name [-]: specifies the name of the output terminal of the Simulink block.
      | - Index [-]: specifies the start position in the output vector sent to the Sensor World
      | - Port dimensions [-]: specifies the width (number of scalars) of the output port
      | - Upload period [s]: specifies the upload period (in seconds) of the port.
      mask Display: port_label('input', 1, PortName)
  RPY : Subsystem  mask(ToSensorWorld){PortName=RPY_Mazda_RX8_1, PortIndex=24, PortWidth=3, TimeStep=1/500}
      mask prompts: PortName "Port Name [-]"; PortIndex "Index [-]"; PortWidth "Port Dimensions [-]"; TimeStep "Upload Period [s]"
      mask help: Sends signal(s) from Simulink to the Sensor World
      mask Help:
      | Sends signal(s) from Simulink to the Sensor World.
      | 
      | - Port Name [-]: specifies the name of the output terminal of the Simulink block.
      | - Index [-]: specifies the start position in the output vector sent to the Sensor World
      | - Port dimensions [-]: specifies the width (number of scalars) of the output port
      | - Upload period [s]: specifies the upload period (in seconds) of the port.
      mask Display: port_label('input', 1, PortName)
  Velocity : Subsystem  mask(ToSensorWorld){PortName=Velocity_Mazda_RX8_1, PortIndex=18, PortWidth=3, TimeStep=1/500}
      mask prompts: PortName "Port Name [-]"; PortIndex "Index [-]"; PortWidth "Port Dimensions [-]"; TimeStep "Upload Period [s]"
      mask help: Sends signal(s) from Simulink to the Sensor World
      mask Help:
      | Sends signal(s) from Simulink to the Sensor World.
      | 
      | - Port Name [-]: specifies the name of the output terminal of the Simulink block.
      | - Index [-]: specifies the start position in the output vector sent to the Sensor World
      | - Port dimensions [-]: specifies the width (number of scalars) of the output port
      | - Upload period [s]: specifies the upload period (in seconds) of the port.
      mask Display: port_label('input', 1, PortName)
  iniBODYAngles wrtVEH [rad] : Constant  Value=[Roll0 Pitch0 0]
  iniVEHAngles wrtGLOB [rad] : Constant  Value=[0 0 Yaw0]
  iniVEHposition wrtGLOB [m] : Constant  Value=[x0 y0 z0]
  state2FullState : Subsystem  mask(PreScan Demux Block:){Mode=Mode}
      mask prompts: Mode "Mask Parameter 1:"
      mask init:
      | if strcmp(Mode,'Positioning')
      |     SwitchMode=1;
      | else
      |     SwitchMode=0;
      | end
      | 
      | set_param([gcb,'/SwitchMode'],'sw',num2str(SwitchMode));
      | set_param([gcb,'/SwitchMode1'],'sw',num2str(SwitchMode));
      mask Display: disp(Mode)
  velRPY : Subsystem  mask(ToSensorWorld){PortName=velRPY_Mazda_RX8_1, PortIndex=27, PortWidth=3, TimeStep=1/500}
      mask prompts: PortName "Port Name [-]"; PortIndex "Index [-]"; PortWidth "Port Dimensions [-]"; TimeStep "Upload Period [s]"
      mask help: Sends signal(s) from Simulink to the Sensor World
      mask Help:
      | Sends signal(s) from Simulink to the Sensor World.
      | 
      | - Port Name [-]: specifies the name of the output terminal of the Simulink block.
      | - Index [-]: specifies the start position in the output vector sent to the Sensor World
      | - Port dimensions [-]: specifies the width (number of scalars) of the output port
      | - Upload period [s]: specifies the upload period (in seconds) of the port.
      mask Display: port_label('input', 1, PortName)
  wires:
  iniVEHAngles wrtGLOB [rad]/1 -> state2FullState/4(iniVEH Angles wrt GLOB axis system [deg])
  iniBODYAngles wrtVEH [rad]/1 -> state2FullState/3(iniBODY Angles wrt VEH axis system [deg])
  iniVEHposition wrtGLOB [m]/1 -> state2FullState/2(ini VEHpos wrt GLOB axis system  [m])
  state2FullState/1(State) -> Demux/1
  State/1 -> state2FullState/1(dx,dy,dz [m/s] R,P,Y  [rad])
  Demux/1 -> Position/1(Y)
  Demux/2 -> Velocity/1(Y)
  Demux/3 -> Acceleration/1(Y)
  Demux/4 -> RPY/1(Y)
  Demux/5 -> velRPY/1(Y)

== system Demo_veDYNA_cs/STATE_Nissan_Cabstar_1 ==
  State : Inport
  Acceleration : Subsystem  mask(ToSensorWorld){PortName=Acceleration_Nissan_Cabstar_1, PortIndex=280, PortWidth=3, TimeStep=1/500}
      mask prompts: PortName "Port Name [-]"; PortIndex "Index [-]"; PortWidth "Port Dimensions [-]"; TimeStep "Upload Period [s]"
      mask help: Sends signal(s) from Simulink to the Sensor World
      mask Help:
      | Sends signal(s) from Simulink to the Sensor World.
      | 
      | - Port Name [-]: specifies the name of the output terminal of the Simulink block.
      | - Index [-]: specifies the start position in the output vector sent to the Sensor World
      | - Port dimensions [-]: specifies the width (number of scalars) of the output port
      | - Upload period [s]: specifies the upload period (in seconds) of the port.
      mask Display: port_label('input', 1, PortName)
  Demux : Demux  Outputs=5
  Position : Subsystem  mask(ToSensorWorld){PortName=Position_Nissan_Cabstar_1, PortIndex=274, PortWidth=3, TimeStep=1/500}
      mask prompts: PortName "Port Name [-]"; PortIndex "Index [-]"; PortWidth "Port Dimensions [-]"; TimeStep "Upload Period [s]"
      mask help: Sends signal(s) from Simulink to the Sensor World
      mask Help:
      | Sends signal(s) from Simulink to the Sensor World.
      | 
      | - Port Name [-]: specifies the name of the output terminal of the Simulink block.
      | - Index [-]: specifies the start position in the output vector sent to the Sensor World
      | - Port dimensions [-]: specifies the width (number of scalars) of the output port
      | - Upload period [s]: specifies the upload period (in seconds) of the port.
      mask Display: port_label('input', 1, PortName)
  RPY : Subsystem  mask(ToSensorWorld){PortName=RPY_Nissan_Cabstar_1, PortIndex=283, PortWidth=3, TimeStep=1/500}
      mask prompts: PortName "Port Name [-]"; PortIndex "Index [-]"; PortWidth "Port Dimensions [-]"; TimeStep "Upload Period [s]"
      mask help: Sends signal(s) from Simulink to the Sensor World
      mask Help:
      | Sends signal(s) from Simulink to the Sensor World.
      | 
      | - Port Name [-]: specifies the name of the output terminal of the Simulink block.
      | - Index [-]: specifies the start position in the output vector sent to the Sensor World
      | - Port dimensions [-]: specifies the width (number of scalars) of the output port
      | - Upload period [s]: specifies the upload period (in seconds) of the port.
      mask Display: port_label('input', 1, PortName)
  Velocity : Subsystem  mask(ToSensorWorld){PortName=Velocity_Nissan_Cabstar_1, PortIndex=277, PortWidth=3, TimeStep=1/500}
      mask prompts: PortName "Port Name [-]"; PortIndex "Index [-]"; PortWidth "Port Dimensions [-]"; TimeStep "Upload Period [s]"
      mask help: Sends signal(s) from Simulink to the Sensor World
      mask Help:
      | Sends signal(s) from Simulink to the Sensor World.
      | 
      | - Port Name [-]: specifies the name of the output terminal of the Simulink block.
      | - Index [-]: specifies the start position in the output vector sent to the Sensor World
      | - Port dimensions [-]: specifies the width (number of scalars) of the output port
      | - Upload period [s]: specifies the upload period (in seconds) of the port.
      mask Display: port_label('input', 1, PortName)
  iniBODYAngles wrtVEH [rad] : Constant  Value=[Roll0 Pitch0 0]
  iniVEHAngles wrtGLOB [rad] : Constant  Value=[0 0 Yaw0]
  iniVEHposition wrtGLOB [m] : Constant  Value=[x0 y0 z0]
  state2FullState : Subsystem  mask(PreScan Demux Block:){Mode=Mode}
      mask prompts: Mode "Mask Parameter 1:"
      mask init:
      | if strcmp(Mode,'Positioning')
      |     SwitchMode=1;
      | else
      |     SwitchMode=0;
      | end
      | 
      | set_param([gcb,'/SwitchMode'],'sw',num2str(SwitchMode));
      | set_param([gcb,'/SwitchMode1'],'sw',num2str(SwitchMode));
      mask Display: disp(Mode)
  velRPY : Subsystem  mask(ToSensorWorld){PortName=velRPY_Nissan_Cabstar_1, PortIndex=286, PortWidth=3, TimeStep=1/500}
      mask prompts: PortName "Port Name [-]"; PortIndex "Index [-]"; PortWidth "Port Dimensions [-]"; TimeStep "Upload Period [s]"
      mask help: Sends signal(s) from Simulink to the Sensor World
      mask Help:
      | Sends signal(s) from Simulink to the Sensor World.
      | 
      | - Port Name [-]: specifies the name of the output terminal of the Simulink block.
      | - Index [-]: specifies the start position in the output vector sent to the Sensor World
      | - Port dimensions [-]: specifies the width (number of scalars) of the output port
      | - Upload period [s]: specifies the upload period (in seconds) of the port.
      mask Display: port_label('input', 1, PortName)
  wires:
  iniVEHAngles wrtGLOB [rad]/1 -> state2FullState/4(iniVEH Angles wrt GLOB axis system [deg])
  iniBODYAngles wrtVEH [rad]/1 -> state2FullState/3(iniBODY Angles wrt VEH axis system [deg])
  iniVEHposition wrtGLOB [m]/1 -> state2FullState/2(ini VEHpos wrt GLOB axis system  [m])
  state2FullState/1(State) -> Demux/1
  State/1 -> state2FullState/1(dx,dy,dz [m/s] R,P,Y  [rad])
  Demux/1 -> Position/1(Y)
  Demux/2 -> Velocity/1(Y)
  Demux/3 -> Acceleration/1(Y)
  Demux/4 -> RPY/1(Y)
  Demux/5 -> velRPY/1(Y)

== system Demo_veDYNA_cs/SetActuators ==
  Data Store Read : DataStoreRead  DataStoreName=SimCoreActuators  SampleTime=0
  SendActuators : S-Function  FunctionName=SendActuatorsBlock  Parameters=TimeStep,NrOfActuators  EnableBusSupport=off  mask(SendActuatorsBlock){TimeStep=TimeStep, NrOfActuators=NrOfActuators}
      mask prompts: TimeStep "Time step [s]"; NrOfActuators "Numer of actuator values"
      mask help: Sends all actuator values to the simulation core
  dummy : Outport
  wires:
  SendActuators/1 -> dummy/1
  Data Store Read/1 -> SendActuators/1
